simulink model "Sim6_OrthogonalArm_Z_OA"  (R2021a)
settings: Solver=VariableStepAuto  StartTime=0.0  StopTime=Inf  RelTol=1e-3
InitFcn:
  | run('settingParams.m')
  | %GUI = evalin('base','GUI_handle');
undefined symbols (not defined in the file or in its folder): ArmInitPos, dt
libraries: robotlib x3
CloseFcn:
  | %set(findobj(GUI,'Tag','open_sim6'),'Value','Close');
  | %set(findobj(GUI,'Tag','open_sim6'),'Enable','on');
  | %set(findobj(GUI,'Tag','start_sim6'),'Value','Stop');
  | %set(findobj(GUI,'Tag','start_sim6'),'Enable','off');
  | %set(findobj(GUI,'Tag','Lamp_sim6'),'Color',[0.8 0.8 0.8]);
settings Model: Creator=shdet  LastModifiedBy=tomat
settings SolverCC: AlgebraicLoopSolver=TrustRegion
settings DebuggingCC: SFMachineParentedDataDiag=warning
settings SFSimCC: CustomCodeUndefinedFunction=UseInterfaceOnly

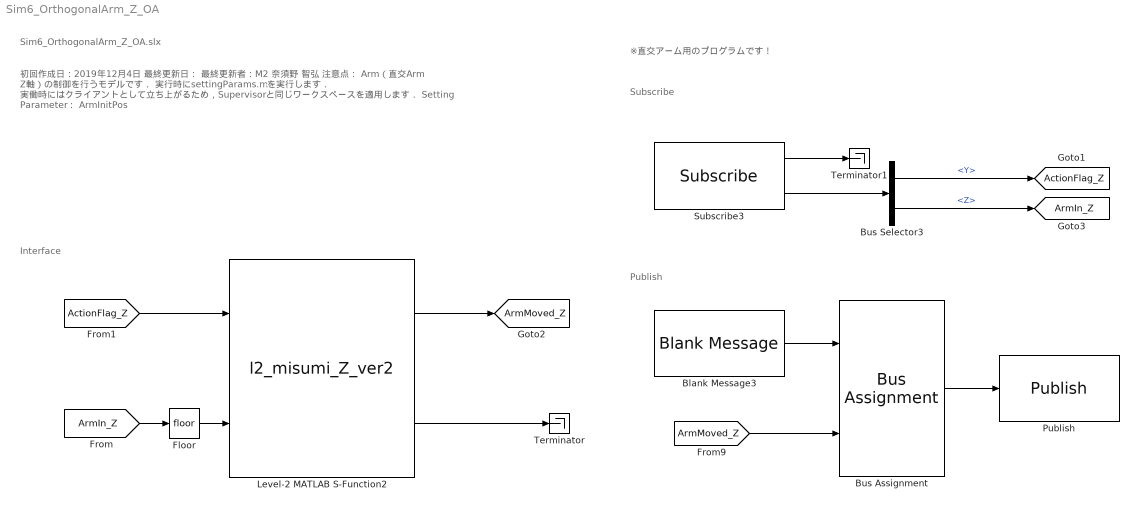
== system Sim6_OrthogonalArm_Z_OA ==
  note: Publish
  note: Sim6_OrthogonalArm_Z_OA.slx
  note: Subscribe
  note: ※直交アーム用のプログラムです！
  note: 初回作成日：2019年12月4日
      | 最終更新日：
      | 最終更新者：M2 奈須野 智弘
      | 注意点：
      | Arm（直交Arm Z軸）の制御を行うモデルです．
      | 実行時にsettingParams.mを実行します．
      | 実働時にはクライアントとして立ち上がるため，Supervisorと同じワークスペースを適用します．
      |
      | Setting Parameter：
      | ArmInitPos
  note: Interface
  Blank Message3 : robotlib/Blank Message  messageClass=Message  entityType=geometry_msgs/TwistStamped  messageType=geometry_msgs/TwistStamped  SampleTime=inf  legacyBusStruct=off
  Bus Assignment : BusAssignment  AssignedSignals=Twist.Linear.X
  Bus Selector3 : BusSelector  OutputSignals=Twist.Linear.Y,Twist.Linear.Z
  Floor : Rounding
  Level-2 MATLAB S-Function2 : M-S-Function  FunctionName=l2_misumi_Z_ver2  Parameters=comport, boundrate, initPos  mask{comport='COM13', boundrate=115200, initPos=ArmInitPos(3)}
      mask prompts: comport "Port Number"; boundrate "Bound Rate"; initPos "Init Position"
      mask Display:
      | disp('Misumi zActuator Control Block');
      | port_label('input',1,'Act.Flag');
      | port_label('input',2,'Target Pos');
      | port_label('output',1,'Moved State');
      | port_label('output',2,'Current State');
  Publish : robotlib/Publish  topicSource=Specify your own  topic=/ARM_Z_S  messageType=geometry_msgs/TwistStamped  legacyBusStruct=off  messageQueueLength=1
  Subscribe3 : robotlib/Subscribe  topicSource=Specify your own  topic=/ARM_S  messageType=geometry_msgs/TwistStamped  SampleTime=dt  legacyBusStruct=off  messageQueueLength=1
  Terminator : Terminator
  Terminator1 : Terminator
  tag scope: ActionFlag_Z=global, ArmIn_Z=global, ArmMoved_Z=global
  wires:
  Bus Selector3/1 -> [ActionFlag_Z]  "<Y>"
  Subscribe3/2 -> Bus Selector3/1
  Subscribe3/1 -> Terminator1/1
  [ArmMoved_Z] -> Bus Assignment/2
  Blank Message3/1 -> Bus Assignment/1
  Bus Assignment/1 -> Publish/1
  [ArmIn_Z] -> Floor/1
  Level-2 MATLAB S-Function2/2 -> Terminator/1
  [ActionFlag_Z] -> Level-2 MATLAB S-Function2/1
  Level-2 MATLAB S-Function2/1 -> [ArmMoved_Z]
  Floor/1 -> Level-2 MATLAB S-Function2/2
  Bus Selector3/2 -> [ArmIn_Z]  "<Z>"
